simulink model "NavV1_0421_2017a"  (R2017a)
settings: Solver=FixedStepAuto  StartTime=0.0  StopTime=589  FixedStep=dt  RelTol=1e-3
values from neighbouring files (symbols this model uses):
  dt = 0.01    [initNavigation.m]
  g0 = 9.798    [initNavigation.m]
  GPSdt = 0.1    [initNavigation.m]
undefined symbols (not defined in the file or in its folder): DiscIntNeverNeededParam, magnitude, param
libraries: simulink x14, simulink_extras x11, sharedtransform x7, aerolibtransform2 x4, dspstat3 x4, dspsolvers x2, aerolibconvert2 x1
(part 1 of 2)
settings Model: Creator=Ye Xiaoyu  LastModifiedBy=Ye Xiaoyu
settings DataIOCC: ReturnWorkspaceOutputs=on
settings DebuggingCC: SFMachineParentedDataDiag=error
settings SFSimCC: SimUseLocalCustomCode=on
settings RTWCC: RTWUseLocalCustomCode=on

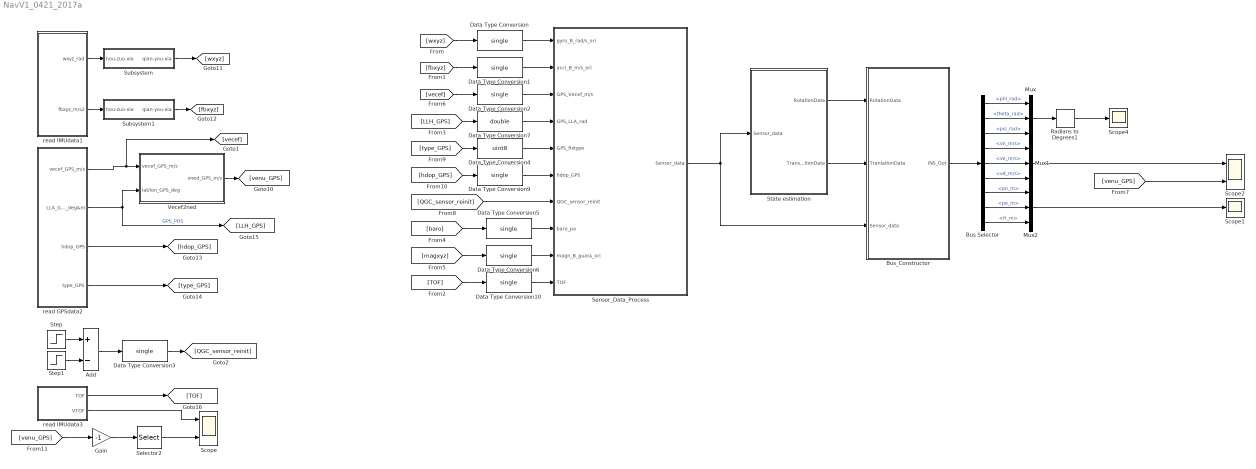
== system NavV1_0421_2017a ==
  Add : Sum  Inputs=+-
  Bus Selector : BusSelector  OutputSignals=phi_rad,theta_rad,psi_rad,vn_m/s,ve_m/s,vd_m/s,pn_m,pe_m,H_m
  Bus_Constructor : Subsystem
  Data Type Conversion{,1..3,5..6,9..10} (8 alike) : DataTypeConversion  OutDataTypeStr=single
  Data Type Conversion4 : DataTypeConversion  OutDataTypeStr=uint8
  Data Type Conversion7 : DataTypeConversion  OutDataTypeStr=double
  Gain : Gain  Gain=-1
  Mux : Mux  Inputs=3
  Mux1 : Mux  Inputs=3
  Mux2 : Mux  Inputs=3
  Radians to Degrees1 : simulink_extras/Transformations/Radians to Degrees
  Scope : Scope  NumInputPorts=2
  Scope1 : Scope
  Scope2 : Scope  NumInputPorts=2
  Scope4 : Scope
  Selector2 : Selector  InputPortWidth=3  IndexOptions=Index vector (dialog)  Indices=[3]  OutputSizes=1
  Sensor_Data_Process : Subsystem
  State estimation : Subsystem
  Step : Step  Time=5  SampleTime=0
  Step1 : Step  Time=5.005  SampleTime=0
  Subsystem : Subsystem
  Subsystem1 : Subsystem
  Vecef2ned : Subsystem
  read GPSdata2 : Subsystem
  read IMUdata1 : Subsystem
  read IMUdata3 : Subsystem
  wires:
  [wxyz] -> Data Type Conversion/1
  [fbxyz] -> Data Type Conversion1/1
  read GPSdata2/1(vecef_GPS_m/s) -> [vecef], Vecef2ned/1(vecef_GPS_m/s)
  [type_GPS] -> Data Type Conversion4/1
  Data Type Conversion/1 -> Sensor_Data_Process/1(gyro_B_rad/s_ori)
  Data Type Conversion1/1 -> Sensor_Data_Process/2(accl_B_m/s_ori)
  Data Type Conversion2/1 -> Sensor_Data_Process/3(GPS_Vecef_m/s)
  [LLH_GPS] -> Data Type Conversion7/1
  Data Type Conversion4/1 -> Sensor_Data_Process/5(GPS_fixtype)
  [QGC_sensor_reinit] -> Sensor_Data_Process/7(QGC_sensor_reinit)
  [baro] -> Data Type Conversion5/1
  [magxyz] -> Data Type Conversion6/1
  Sensor_Data_Process/1(Sensor_data) -> Bus_Constructor/3(Sensor_data), State estimation/1(Sensor_data)
  Data Type Conversion5/1 -> Sensor_Data_Process/8(baro_pa)
  Data Type Conversion6/1 -> Sensor_Data_Process/9(magn_B_guass_ori)
  Data Type Conversion7/1 -> Sensor_Data_Process/4(GPS_LLA_rad)
  Mux1/1 -> Scope2/1
  [venu_GPS] -> Scope2/2
  Mux2/1 -> Scope1/1
  read IMUdata1/2(fbxyz_m/s2) -> Subsystem1/1(hou-zuo-xia)
  read IMUdata1/1(wxyz_rad) -> Subsystem/1(hou-zuo-xia)
  read GPSdata2/2(LLA_GPS_deg&m) -> [LLH_GPS], Vecef2ned/2(lat/lon_GPS_deg)  "GPS_POS"
  Vecef2ned/1(vned_GPS_m/s) -> [venu_GPS]
  read GPSdata2/3(hdop_GPS) -> [hdop_GPS]
  read GPSdata2/4(type_GPS) -> [type_GPS]
  Data Type Conversion9/1 -> Sensor_Data_Process/6(hdop_GPS)
  [hdop_GPS] -> Data Type Conversion9/1
  Subsystem/1(qian-you-xia) -> [wxyz]
  Subsystem1/1(qian-you-xia) -> [fbxyz]
  read IMUdata3/1(TOF) -> [TOF]
  [TOF] -> Data Type Conversion10/1
  Data Type Conversion10/1 -> Sensor_Data_Process/10(TOF)
  read IMUdata3/2(VTOF) -> Scope/1
  [venu_GPS] -> Gain/1
  Selector2/1 -> Scope/2
  Gain/1 -> Selector2/1
  State estimation/1(RotationData) -> Bus_Constructor/1(RotationData)
  State estimation/2(TranslationData) -> Bus_Constructor/2(TranlationData)
  Bus_Constructor/1(INS_Out) -> Bus Selector/1
  Bus Selector/1 -> Mux/1  "<phi_rad>"
  Bus Selector/2 -> Mux/2  "<theta_rad>"
  Bus Selector/3 -> Mux/3  "<psi_rad>"
  Bus Selector/4 -> Mux1/1  "<vn_m/s>"
  Bus Selector/5 -> Mux1/2  "<ve_m/s>"
  Bus Selector/6 -> Mux1/3  "<vd_m/s>"
  Bus Selector/7 -> Mux2/1  "<pn_m>"
  Bus Selector/8 -> Mux2/2  "<pe_m>"
  Bus Selector/9 -> Mux2/3  "<H_m>"
  Mux/1 -> Radians to Degrees1/1
  Radians to Degrees1/1 -> Scope4/1
  [vecef] -> Data Type Conversion2/1
  Step/1 -> Add/1
  Add/1 -> Data Type Conversion3/1
  Step1/1 -> Add/2
  Data Type Conversion3/1 -> [QGC_sensor_reinit]

== system NavV1_0421_2017a/Bus_Constructor ==
  RotationData : Inport
  TranlationData : Inport  Port=2
  Sensor_data : Inport  Port=3
  Bus Creator : BusCreator  Inputs=13
  Bus Selector1 : BusSelector  OutputSignals=vn_m/s,ve_m/s,vd_m/s,pn_m,pe_m,H_m
  Bus Selector2 : BusSelector  OutputSignals=IMU_Data.gyro_B_rad/s_LPF,IMU_Data.accl_B_m/s2_LPF,QGC_sensor_reinit
  Rotation_output : Subsystem
  Signal Copy : SignalConversion  OverrideOpt=off
  Signal Copy2 : SignalConversion  OverrideOpt=off
  INS_Out : Outport
  wires:
  Signal Copy/1 -> Bus Selector2/1
  Sensor_data/1 -> Signal Copy/1
  Bus Selector2/1 -> Bus Creator/1  "<gyro_B_rad/s_LPF>"
  Bus Selector2/2 -> Bus Creator/2  "<accl_B_m/s2_LPF>"
  Bus Selector2/3 -> Bus Creator/3  "<QGC_sensor_reinit>"
  TranlationData/1 -> Signal Copy2/1
  Signal Copy2/1 -> Bus Selector1/1
  Bus Selector1/1 -> Bus Creator/4  "<vn_m/s>"
  Bus Selector1/2 -> Bus Creator/5  "<ve_m/s>"
  Bus Selector1/3 -> Bus Creator/6  "<vd_m/s>"
  Bus Selector1/4 -> Bus Creator/7  "<pn_m>"
  Bus Selector1/5 -> Bus Creator/8  "<pe_m>"
  Bus Selector1/6 -> Bus Creator/9  "<H_m>"
  RotationData/1 -> Rotation_output/1(RotationData)
  Rotation_output/1(<q_update>) -> Bus Creator/10
  Rotation_output/2(phi_rad) -> Bus Creator/11
  Rotation_output/3(theta_rad) -> Bus Creator/12
  Rotation_output/4(psi_rad) -> Bus Creator/13
  Bus Creator/1 -> INS_Out/1

== system NavV1_0421_2017a/Sensor_Data_Process ==
  gyro_B_rad/s_ori : Inport
  accl_B_m/s_ori : Inport  Port=2
  GPS_Vecef_m/s : Inport  Port=3
  GPS_LLA_rad : Inport  Port=4
  GPS_fixtype : Inport  Port=5
  hdop_GPS : Inport  Port=6
  QGC_sensor_reinit : Inport  Port=7
  baro_pa : Inport  Port=8
  magn_B_guass_ori : Inport  Port=9
  TOF : Inport  Port=10
  Bus Creator : BusCreator  Inputs=6
  GPS_Data_Process : Subsystem
  IMU_Data_Process : Subsystem
  Magn_Data_Process : Subsystem
  QGC_sensor_reinit1 : InportShadow  Port=7
  TOF_Data_Process : Subsystem
  baro_Data_Process : Subsystem
  Sensor_data : Outport
  wires:
  QGC_sensor_reinit/1 -> baro_Data_Process/2(QGC_sensor_reinit), GPS_Data_Process/5(QGC_sensor_reinit)  "QGC_sensor_reinit"
  GPS_Data_Process/1(GPS_Data) -> Bus Creator/2  "GPS_Data"
  IMU_Data_Process/1(IMU_Data) -> Bus Creator/1  "IMU_Data"
  baro_Data_Process/1(BARO_Data) -> Bus Creator/3  "BARO_Data"
  gyro_B_rad/s_ori/1 -> IMU_Data_Process/1(gyro_B_rad/s_ori)
  Magn_Data_Process/1(MAGN_Data) -> Bus Creator/4  "MAGN_Data"
  baro_pa/1 -> baro_Data_Process/1(baro)
  accl_B_m/s_ori/1 -> IMU_Data_Process/2(accl_B_m/s_ori)
  magn_B_guass_ori/1 -> Magn_Data_Process/1(magn_B_guass_ori)
  GPS_LLA_rad/1 -> GPS_Data_Process/2(GPS_LLA_rad)
  GPS_Vecef_m/s/1 -> GPS_Data_Process/1(GPS_Vecef_m/s)
  GPS_fixtype/1 -> GPS_Data_Process/3(GPS_fixtype)
  Bus Creator/1 -> Sensor_data/1
  hdop_GPS/1 -> GPS_Data_Process/4(hdop_GPS)
  QGC_sensor_reinit1/1 -> Bus Creator/6  "QGC_sensor_reinit"
  TOF/1 -> TOF_Data_Process/1(TOF_mm_ori)
  TOF_Data_Process/1(TOF_Data) -> Bus Creator/5

== system NavV1_0421_2017a/State estimation ==
  Sensor_data : Inport
  AHRS : Subsystem
  Bus Selector : BusSelector  OutputSignals=QGC_sensor_reinit,IMU_Data.accl_B_m/s2_LPF,MAGN_Data,GPS_Data
  Sensor_data1 : InportShadow
  Sensor_data2 : InportShadow
  Translation_estimate : Subsystem
  RotationData : Outport
  TranslationData : Outport  Port=2
  wires:
  Sensor_data/1 -> Bus Selector/1
  Bus Selector/1 -> AHRS/1(<QGC_sensor_reinit>)  "<QGC_sensor_reinit>"
  Bus Selector/2 -> AHRS/2(<accl_B_m/s2_LPF>)  "<accl_B_m/s2_LPF>"
  Bus Selector/3 -> AHRS/3(<MAGN_Data>)  "<MAGN_Data>"
  Bus Selector/4 -> AHRS/4(<GPS_Data>)  "<GPS_Data>"
  Sensor_data1/1 -> AHRS/5(Sensor_data)
  AHRS/1(RotationData) -> RotationData/1, Translation_estimate/1(RotationData)
  Sensor_data2/1 -> Translation_estimate/2(Sensor_data)
  Translation_estimate/1(TranslationData) -> TranslationData/1

== system NavV1_0421_2017a/Subsystem ==
  hou-zuo-xia : Inport
  Demux : Demux  Outputs=3
  Gain : Gain  Gain=-1
  Gain1 : Gain  Gain=-1
  Mux : Mux  Inputs=3
  qian-you-xia : Outport
  wires:
  Mux/1 -> qian-you-xia/1
  Gain1/1 -> Mux/2
  Demux/3 -> Mux/3
  Gain/1 -> Mux/1
  hou-zuo-xia/1 -> Demux/1
  Demux/1 -> Gain/1
  Demux/2 -> Gain1/1

== system NavV1_0421_2017a/Subsystem1 ==
  hou-zuo-xia : Inport
  Demux : Demux  Outputs=3
  Gain : Gain  Gain=-1
  Gain1 : Gain  Gain=-1
  Mux : Mux  Inputs=3
  qian-you-xia : Outport
  wires:
  Demux/2 -> Gain1/1
  Demux/1 -> Gain/1
  hou-zuo-xia/1 -> Demux/1
  Gain/1 -> Mux/1
  Demux/3 -> Mux/3
  Gain1/1 -> Mux/2
  Mux/1 -> qian-you-xia/1

== system NavV1_0421_2017a/Vecef2ned ==
  vecef_GPS_m/s : Inport
  lat/lon_GPS_deg : Inport  Port=2
  Direction Cosine Matrix ECEF to NED : aerolibtransform2/Direction Cosine Matrix ECEF to NED
      settings: SourceProductBaseCode=AE
  Product : Product  Multiplication=Matrix(*)
  Radians to Degrees : simulink_extras/Transformations/Radians to Degrees
  Selector2 : Selector  InputPortWidth=3  IndexOptions=Index vector (dialog)  Indices=[1 2]  OutputSizes=1
  vned_GPS_m/s : Outport
  wires:
  Direction Cosine Matrix ECEF to NED/1 -> Product/1
  vecef_GPS_m/s/1 -> Product/2
  lat/lon_GPS_deg/1 -> Selector2/1
  Product/1 -> vned_GPS_m/s/1
  Selector2/1 -> Radians to Degrees/1
  Radians to Degrees/1 -> Direction Cosine Matrix ECEF to NED/1

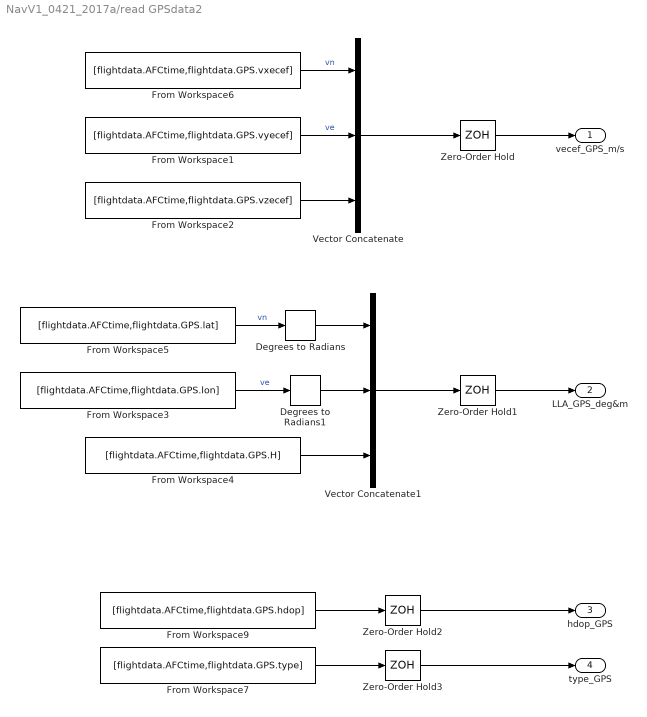
== system NavV1_0421_2017a/read GPSdata2 ==
  Degrees to Radians : simulink_extras/Transformations/Degrees to Radians
  Degrees to Radians1 : simulink_extras/Transformations/Degrees to Radians
  From Workspace1 : FromWorkspace  VariableName=[flightdata.AFCtime,flightdata.GPS.vyecef]
  From Workspace2 : FromWorkspace  VariableName=[flightdata.AFCtime,flightdata.GPS.vzecef]
  From Workspace3 : FromWorkspace  VariableName=[flightdata.AFCtime,flightdata.GPS.lon]
  From Workspace4 : FromWorkspace  VariableName=[flightdata.AFCtime,flightdata.GPS.H]
  From Workspace5 : FromWorkspace  VariableName=[flightdata.AFCtime,flightdata.GPS.lat]
  From Workspace6 : FromWorkspace  VariableName=[flightdata.AFCtime,flightdata.GPS.vxecef]
  From Workspace7 : FromWorkspace  VariableName=[flightdata.AFCtime,flightdata.GPS.type]
  From Workspace9 : FromWorkspace  VariableName=[flightdata.AFCtime,flightdata.GPS.hdop]
  Vector Concatenate : Concatenate  NumInputs=3
  Vector Concatenate1 : Concatenate  NumInputs=3
  Zero-Order Hold{,1..3} (4 alike) : ZeroOrderHold  SampleTime=GPSdt
  vecef_GPS_m/s : Outport
  LLA_GPS_deg&m : Outport  Port=2
  hdop_GPS : Outport  Port=3
  type_GPS : Outport  Port=4
  wires:
  Zero-Order Hold/1 -> vecef_GPS_m/s/1
  Zero-Order Hold1/1 -> LLA_GPS_deg&m/1
  From Workspace6/1 -> Vector Concatenate/1  "vn"
  From Workspace1/1 -> Vector Concatenate/2  "ve"
  From Workspace2/1 -> Vector Concatenate/3
  From Workspace5/1 -> Degrees to Radians/1  "vn"
  From Workspace3/1 -> Degrees to Radians1/1  "ve"
  From Workspace4/1 -> Vector Concatenate1/3
  Vector Concatenate/1 -> Zero-Order Hold/1
  Vector Concatenate1/1 -> Zero-Order Hold1/1
  From Workspace7/1 -> Zero-Order Hold3/1
  Zero-Order Hold2/1 -> hdop_GPS/1
  From Workspace9/1 -> Zero-Order Hold2/1
  Zero-Order Hold3/1 -> type_GPS/1
  Degrees to Radians/1 -> Vector Concatenate1/1
  Degrees to Radians1/1 -> Vector Concatenate1/2

== system NavV1_0421_2017a/read IMUdata1 ==
  note: 后-左-下
  Degrees to Radians1 : simulink_extras/Transformations/Degrees to Radians
  From Workspace1 : FromWorkspace  VariableName=[flightdata.AFCtime,flightdata.IMUADIS16507.wx]
  From Workspace10 : FromWorkspace  VariableName=[flightdata.AFCtime,flightdata.IMUADIS16507.wy]
  From Workspace2 : FromWorkspace  VariableName=[flightdata.AFCtime,flightdata.IMUADIS16507.wz]
  From Workspace3 : FromWorkspace  VariableName=[flightdata.AFCtime,flightdata.IMUADIS16507.fbx]
  From Workspace4 : FromWorkspace  VariableName=[flightdata.AFCtime,flightdata.IMUADIS16507.fby]
  From Workspace5 : FromWorkspace  VariableName=[flightdata.AFCtime,flightdata.IMUADIS16507.fbz]
  Scope : Scope
  Vector Concatenate : Concatenate  NumInputs=3
  Vector Concatenate1 : Concatenate  NumInputs=3
  Zero-Order Hold : ZeroOrderHold  SampleTime=dt
  Zero-Order Hold1 : ZeroOrderHold  SampleTime=dt
  wxyz_rad : Outport
  fbxyz_m/s2 : Outport  Port=2
  wires:
  Degrees to Radians1/1 -> Zero-Order Hold/1
  Zero-Order Hold1/1 -> fbxyz_m/s2/1
  Zero-Order Hold/1 -> wxyz_rad/1
  From Workspace1/1 -> Vector Concatenate/1
  From Workspace10/1 -> Vector Concatenate/2
  From Workspace2/1 -> Vector Concatenate/3
  Vector Concatenate/1 -> Scope/1, Degrees to Radians1/1
  From Workspace3/1 -> Vector Concatenate1/1
  From Workspace4/1 -> Vector Concatenate1/2
  From Workspace5/1 -> Vector Concatenate1/3
  Vector Concatenate1/1 -> Zero-Order Hold1/1

== system NavV1_0421_2017a/read IMUdata3 ==
  note: 后-左-下
  Data Type Conversion : DataTypeConversion  OutDataTypeStr=single
  From Workspace1 : FromWorkspace  VariableName=[flightdata.AFCtime,flightdata.TOF.dist]
  From Workspace10 : FromWorkspace  VariableName=[flightdata.AFCtime,flightdata.TOF.Inten]
  From Workspace2 : FromWorkspace  VariableName=[flightdata.AFCtime,flightdata.TOF.sts]
  Gain : Gain  Gain=0.01
  Scope : Scope
  Scope1 : Scope  NumInputPorts=3
  TD_baro : Subsystem
  Vector Concatenate : Concatenate  NumInputs=3
  Zero-Order Hold : ZeroOrderHold  SampleTime=dt
  TOF : Outport
  VTOF : Outport  Port=2
  wires:
  Vector Concatenate/1 -> Zero-Order Hold/1, Scope/1
  From Workspace2/1 -> Vector Concatenate/3
  From Workspace10/1 -> Vector Concatenate/2
  From Workspace1/1 -> Scope1/1, Data Type Conversion/1, Vector Concatenate/1
  Zero-Order Hold/1 -> TOF/1
  TD_baro/1(vH_baro_TD) -> VTOF/1, Scope1/2  "vH_baro_m/s_TD"
  TD_baro/2(H_baro_TD) -> Scope1/3  "H_baro_TD"
  Data Type Conversion/1 -> Gain/1
  Gain/1 -> TD_baro/1(H_baro)

== system NavV1_0421_2017a/Bus_Constructor/Rotation_output ==
  RotationData : Inport
  Bus Selector3 : BusSelector  OutputSignals=q_update
  Data Type Conversion11 : DataTypeConversion  OutDataTypeStr=single
  Data Type Conversion12 : DataTypeConversion  OutDataTypeStr=double
  Demux : Demux  Outputs=3
  Quaternions to Rotation Angles1 : sharedtransform/Quaternions to Rotation Angles  rotationOrder=ZYX
      settings: SourceProductBaseCode=AE,PW,DR,MT,UV,VE
  Signal Copy1 : SignalConversion  OverrideOpt=off
  <q_update> : Outport
  phi_rad : Outport  Port=2
  theta_rad : Outport  Port=3
  psi_rad : Outport  Port=4
  wires:
  Quaternions to Rotation Angles1/1 -> Data Type Conversion11/1
  Bus Selector3/1 -> <q_update>/1, Data Type Conversion12/1  "<q_update>"
  Signal Copy1/1 -> Bus Selector3/1
  RotationData/1 -> Signal Copy1/1
  Data Type Conversion12/1 -> Quaternions to Rotation Angles1/1
  Demux/1 -> psi_rad/1  "psi_rad"
  Data Type Conversion11/1 -> Demux/1
  Demux/2 -> theta_rad/1  "theta_rad"
  Demux/3 -> phi_rad/1  "phi_rad"

== system NavV1_0421_2017a/Sensor_Data_Process/GPS_Data_Process ==
  note: GPS_fixtype:
      | 0: 定位不可用或无效
      | 1:单点定位
      | 2:伪距差分
      | 4:RTK固定解
  GPS_Vecef_m/s : Inport
  GPS_LLA_rad : Inport  Port=2
  GPS_fixtype : Inport  Port=3
  hdop_GPS : Inport  Port=4
  QGC_sensor_reinit : Inport  Port=5
  Bus Creator : BusCreator  Inputs=13
  Demux : Demux  Outputs=3
  Demux1 : Demux  Outputs=3
  Demux3 : Demux  Outputs=3
  LLA2NED : Subsystem
  Subsystem : Subsystem
  GPS_Data : Outport
  wires:
  Bus Creator/1 -> GPS_Data/1
  Demux3/3 -> Bus Creator/3  "H_gps"
  Demux/3 -> Bus Creator/9  "vd_gps"
  Demux/1 -> Bus Creator/7  "vn_gps"
  GPS_LLA_rad/1 -> Demux3/1, LLA2NED/1(gps_LLA_rad)
  Demux/2 -> Bus Creator/8  "ve_gps"
  Demux3/2 -> Bus Creator/2  "lon_gps"
  Demux3/1 -> Bus Creator/1  "lat_gps"
  GPS_fixtype/1 -> Bus Creator/12  "fixtype_gps"
  QGC_sensor_reinit/1 -> LLA2NED/3(QGC_sensor_reinit)  "QGC_sensor_reinit"
  LLA2NED/1("gpsposNEDout ") -> Demux1/1
  Demux1/1 -> Bus Creator/4  "pos_N_gps"
  Demux1/2 -> Bus Creator/5  "pos_E_gps"
  Demux1/3 -> Bus Creator/6  "pos_D_gps"
  GPS_Vecef_m/s/1 -> LLA2NED/2(GPS_Vecef_m/s)
  LLA2NED/2(gpsvNEDout) -> Subsystem/1(Vned), Demux/1
  Subsystem/1(heading_GPS_rad) -> Bus Creator/10  "heading_GPS_rad"
  Subsystem/2(heading_GPS_valid) -> Bus Creator/11  "heading_GPS_valid"
  hdop_GPS/1 -> Bus Creator/13  "hdop_GPS"

== system NavV1_0421_2017a/Sensor_Data_Process/IMU_Data_Process ==
  gyro_B_rad/s_ori : Inport
  accl_B_m/s_ori : Inport  Port=2
  Bus Creator : BusCreator  Inputs=2
  accl_preprocessing : Subsystem
  gyro_preprocessing : Subsystem
  IMU_Data : Outport  PortDimensions=6
  wires:
  Bus Creator/1 -> IMU_Data/1
  gyro_preprocessing/1(gyro_B_rad/s_LPF) -> Bus Creator/1  "gyro_B_rad/s_LPF"
  accl_B_m/s_ori/1 -> accl_preprocessing/1(accl_B_m/s_ori)
  accl_preprocessing/1(accl_B_m/s2_LPF) -> Bus Creator/2  "accl_B_m/s2_LPF"
  gyro_B_rad/s_ori/1 -> gyro_preprocessing/1(gyro_B_rad/s_ori)

== system NavV1_0421_2017a/Sensor_Data_Process/Magn_Data_Process ==
  magn_B_guass_ori : Inport
  gyro_preprocessing : Subsystem
  MAGN_Data : Outport
  wires:
  magn_B_guass_ori/1 -> gyro_preprocessing/1(gyro_B_rad/s_ori)
  gyro_preprocessing/1(gyro_B_rad/s_LPF) -> MAGN_Data/1  "gyro_B_rad/s_LPF"

== system NavV1_0421_2017a/Sensor_Data_Process/TOF_Data_Process ==
  TOF_mm_ori : Inport
  Bus Creator1 : BusCreator  Inputs=4
  Data Type Conversion : DataTypeConversion  OutDataTypeStr=uint8
  Demux : Demux  Outputs=3
  Gain : Gain  Gain=0.01
  TD_baro : Subsystem
  TOF_Data : Outport
  wires:
  TD_baro/2(H_TOF_TD) -> Bus Creator1/2  "H_TOF_TD"
  Demux/3 -> Data Type Conversion/1  "TOF_sts"
  Demux/1 -> Gain/1
  TOF_mm_ori/1 -> Demux/1
  Demux/2 -> Bus Creator1/3  "TOF_Inten"
  Bus Creator1/1 -> TOF_Data/1  "TOF_Data"
  TD_baro/1(vH_TOF_TD) -> Bus Creator1/1  "vH_TOF_m/s_TD"
  Gain/1 -> TD_baro/1(H_TOF)  "TOF_Dist_m"
  Data Type Conversion/1 -> Bus Creator1/4  "TOF_sts"

== system NavV1_0421_2017a/Sensor_Data_Process/baro_Data_Process ==
  baro : Inport
  QGC_sensor_reinit : Inport  Port=2
  Bus Creator : BusCreator  Inputs=2
  Pressure2Height : Subsystem
  Scope : Scope  NumInputPorts=2
  Sum : Sum  Inputs=|+-
  TD_baro : Subsystem
  reinit_baro0 : Subsystem
  BARO_Data : Outport  PortDimensions=2
  wires:
  Sum/1 -> Bus Creator/2  "H_baro_m_TD"
  TD_baro/1(vH_baro_TD) -> Scope/1, Bus Creator/1  "vH_baro_m/s_TD"
  baro/1 -> Pressure2Height/1(baro)
  Bus Creator/1 -> BARO_Data/1
  Pressure2Height/1(H_baro) -> TD_baro/1(H_baro)
  QGC_sensor_reinit/1 -> reinit_baro0/1(QGC_sensor_reinit)
  TD_baro/2(H_baro_TD) -> Scope/2, Sum/1, reinit_baro0/2(Data)  "H_baro_TD"
  reinit_baro0/1(dataout) -> Sum/2

== system NavV1_0421_2017a/State estimation/AHRS ==
  <QGC_sensor_reinit> : Inport  PortDimensions=1
  <accl_B_m/s2_LPF> : Inport  Port=2  PortDimensions=3
  <MAGN_Data> : Inport  Port=3  PortDimensions=3
  <GPS_Data> : Inport  Port=4
  Sensor_data : Inport  Port=5
  <QGC_sensor_reinit>1 : InportShadow  PortDimensions=1
  AHRS Complementary filter : Subsystem  mask{GPS_accel_kp=0.2, GPS_accel_ki=0, noGPS_accel_kp=0.3, noGPS_accel_ki=0}
      mask prompts: GPS_accel_kp "GPS修正下互补滤波增益kp"; GPS_accel_ki "GPS修正下互补滤波增益Ki"; noGPS_accel_kp "无GPS修正下互补滤波增益kp"; noGPS_accel_ki "无GPS修正下互补滤波增益Ki"
      mask DialogControl DescTextVar Prompt: AHRS Complementary filter
  Bus Selector1 : BusSelector  OutputSignals=IMU_Data.accl_B_m/s2_LPF
  Bus Selector2 : BusSelector  OutputSignals=MAGN_Data
  Init_Q0 : Subsystem
  Scope : Scope
  Sensor_data_1 : InportShadow  Port=5
  att_update : Subsystem
  RotationData : Outport
  wires:
  Sensor_data/1 -> att_update/1(Sensor_data)
  Sensor_data_1/1 -> Bus Selector2/1, Bus Selector1/1
  Bus Selector1/1 -> AHRS Complementary filter/1(fbxyz)  "<accl_B_m/s2_LPF>"
  Bus Selector2/1 -> AHRS Complementary filter/4(magxyz)  "<MAGN_Data>"
  <GPS_Data>/1 -> AHRS Complementary filter/3(GPS_Data)
  <QGC_sensor_reinit>1/1 -> att_update/3(init_flag)
  att_update/1(att_update) -> RotationData/1, AHRS Complementary filter/2(Q_update)
  AHRS Complementary filter/1(w_bias) -> att_update/4(wbias), Scope/1
  <QGC_sensor_reinit>/1 -> Init_Q0/1(U)
  <accl_B_m/s2_LPF>/1 -> Init_Q0/2(accl_B_m/s_LPF)
  <MAGN_Data>/1 -> Init_Q0/3(Magn_B_guess_LPF)
  Init_Q0/1(quat_0) -> att_update/2(quat_0)

== system NavV1_0421_2017a/State estimation/Translation_estimate ==
  RotationData : Inport
  Sensor_data : Inport  Port=2
  Bus Creator : BusCreator  Inputs=2
  Bus Creator2 : BusCreator  Inputs=6
  Demux : Demux  Outputs=2
  Demux1 : Demux  Outputs=2
  Gain : Gain  Gain=-1
  High data source selection : Subsystem
  Rxy_Horizontal_estimation : Subsystem
  Subsystem : Subsystem
  V_Horizontal_estimation : Subsystem
  V_Vertical_estimation : Subsystem
  translate to N : Subsystem
  TranslationData : Outport
  wires:
  Sensor_data/1 -> High data source selection/1(Sensor_data), Subsystem/2(sensor_data), V_Vertical_estimation/2(Sensor_data), Rxy_Horizontal_estimation/3(Sensor_data2), V_Horizontal_estimation/2(Sensor_data2), translate to N/2(Sensor_data)
  RotationData/1 -> translate to N/1(RotationData)
  Rxy_Horizontal_estimation/1(R_n&e) -> Demux1/1
  translate to N/1(accel_Horizontal_predict) -> V_Horizontal_estimation/1(An)
  V_Horizontal_estimation/1(vxy_estimout) -> Demux/1  "v_ne_"
  V_Horizontal_estimation/2(V_n&e) -> Rxy_Horizontal_estimation/1(Vn)
  V_Horizontal_estimation/3(GPS_v_enable) -> Rxy_Horizontal_estimation/2(Enable)
  translate to N/2(accel_Vertical_predict) -> V_Vertical_estimation/1(accel_Vertical_predict)
  V_Vertical_estimation/1(Vh_vertical_eastimate) -> Subsystem/1(Vh_vertical_eastimate), Gain/1  "vh_m/s"
  High data source selection/1(HTOF_vaild_flag) -> Bus Creator/1  "HTOF_vaild"
  High data source selection/2(HGPS_vaild_flag) -> Bus Creator/2  "HGPS_vaild"
  Bus Creator/1 -> Subsystem/3(Vertical_vaild_flag), V_Vertical_estimation/3(Vertical_vaild_flag)
  Subsystem/1(H_estimation) -> Bus Creator2/6  "H_m"
  Demux/1 -> Bus Creator2/1  "vn_m/s"
  Demux/2 -> Bus Creator2/2  "ve_m/s"
  Demux1/1 -> Bus Creator2/4  "pn_m"
  Demux1/2 -> Bus Creator2/5  "pe_m"
  Gain/1 -> Bus Creator2/3  "vd_m/s"
  Bus Creator2/1 -> TranslationData/1

== system NavV1_0421_2017a/read IMUdata3/TD_baro ==
  H_baro : Inport
  Constant1 : Constant  Value=dt  OutDataTypeStr=single
  Constant3 : Constant  Value=0.23  OutDataTypeStr=single
  Constant4 : Constant  Value=1000  OutDataTypeStr=single
  Delay1 : Delay  DelayLength=1  InitialConditionSource=Input port
      settings: InputPortMap=u0,p4
  MATLAB Function2 : MATLAB Function  TreatAsAtomicUnit=on
  Memory : Memory  InheritSampleTime=on
  Scope : Scope  NumInputPorts=3
  vH_baro_TD : Outport
  H_baro_TD : Outport  Port=2
  wires:
  Delay1/1 -> H_baro_TD/1, Scope/3, MATLAB Function2/3("u1 ")
  H_baro/1 -> Delay1/2, MATLAB Function2/2(u0), Scope/1
  Memory/1 -> MATLAB Function2/4("u2 "), vH_baro_TD/1, Scope/2
  Constant3/1 -> MATLAB Function2/5(h)
  Constant1/1 -> MATLAB Function2/1(T)
  Constant4/1 -> MATLAB Function2/6(r)
  MATLAB Function2/1(u1) -> Delay1/1
  MATLAB Function2/2(u2) -> Memory/1

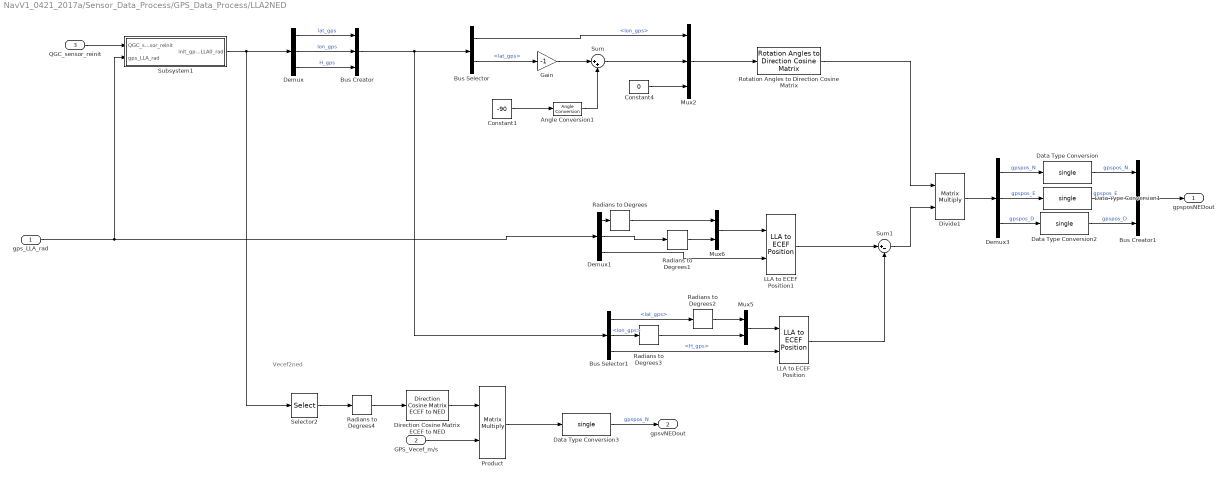
== system NavV1_0421_2017a/Sensor_Data_Process/GPS_Data_Process/LLA2NED ==
  note: Vecef2ned
  gps_LLA_rad : Inport
  GPS_Vecef_m/s : Inport  Port=2
  QGC_sensor_reinit : Inport  Port=3
  Angle Conversion1 : aerolibconvert2/Angle Conversion  IU=deg  OU=rad
  Bus Creator : BusCreator  Inputs=3
  Bus Creator1 : BusCreator  Inputs=3
  Bus Selector : BusSelector  OutputSignals=lon_gps,lat_gps
  Bus Selector1 : BusSelector  OutputSignals=lat_gps,lon_gps,H_gps
  Constant1 : Constant  Value=-90
  Constant4 : Constant  Value=0
  Data Type Conversion{,1..3} (4 alike) : DataTypeConversion  OutDataTypeStr=single
  Demux : Demux  Outputs=3
  Demux1 : Demux  Outputs=3
  Demux3 : Demux  Outputs=3
  Direction Cosine Matrix ECEF to NED : aerolibtransform2/Direction Cosine Matrix ECEF to NED
      settings: SourceProductBaseCode=AE
  Divide1 : Product  Inputs=**  Multiplication=Matrix(*)
  Gain : Gain  Gain=-1
  LLA to ECEF Position : aerolibtransform2/LLA to ECEF Position  R=6378137
  LLA to ECEF Position1 : aerolibtransform2/LLA to ECEF Position  R=6378137
  Mux2 : Mux  Inputs=3
  Mux5 : Mux  Inputs=2
  Mux6 : Mux  Inputs=2
  Product : Product  Multiplication=Matrix(*)
  Radians to Degrees{,1..4} (5 alike) : simulink_extras/Transformations/Radians to Degrees
  Rotation Angles to Direction Cosine Matrix : sharedtransform/Rotation Angles to Direction Cosine Matrix  rotationOrder=ZYX
      settings: SourceProductBaseCode=AE
  Selector2 : Selector  InputPortWidth=3  IndexOptions=Index vector (dialog)  Indices=[1 2]  OutputSizes=1
  Subsystem1 : Subsystem
  Sum : Sum  Inputs=|++
  Sum1 : Sum  Inputs=|+-
  "gpsposNEDout " : Outport
  gpsvNEDout : Outport  Port=2
  wires:
  Bus Creator1/1 -> "gpsposNEDout "/1
  Demux3/3 -> Data Type Conversion2/1  "gpspos_D"
  Demux3/2 -> Data Type Conversion1/1  "gpspos_E"
  Demux3/1 -> Data Type Conversion/1  "gpspos_N"
  Bus Creator/1 -> Bus Selector/1, Bus Selector1/1
  Demux/3 -> Bus Creator/3  "H_gps"
  Demux/2 -> Bus Creator/2  "lon_gps"
  Demux/1 -> Bus Creator/1  "lat_gps"
  Demux1/3 -> LLA to ECEF Position1/2
  Mux6/1 -> LLA to ECEF Position1/1
  Mux5/1 -> LLA to ECEF Position/1
  Gain/1 -> Sum/1
  LLA to ECEF Position1/1 -> Sum1/1
  Constant4/1 -> Mux2/3
  Sum1/1 -> Divide1/2
  Divide1/1 -> Demux3/1
  Demux1/1 -> Radians to Degrees/1
  Mux2/1 -> Rotation Angles to Direction Cosine Matrix/1
  Rotation Angles to Direction Cosine Matrix/1 -> Divide1/1
  Constant1/1 -> Angle Conversion1/1
  LLA to ECEF Position/1 -> Sum1/2
  Demux1/2 -> Radians to Degrees1/1
  Sum/1 -> Mux2/2
  Bus Selector/2 -> Gain/1  "<lat_gps>"
  Bus Selector/1 -> Mux2/1  "<lon_gps>"
  Bus Selector1/1 -> Radians to Degrees2/1  "<lat_gps>"
  Bus Selector1/2 -> Radians to Degrees3/1  "<lon_gps>"
  Bus Selector1/3 -> LLA to ECEF Position/2  "<H_gps>"
  gps_LLA_rad/1 -> Subsystem1/2(gps_LLA_rad), Demux1/1
  Radians to Degrees/1 -> Mux6/1
  Radians to Degrees1/1 -> Mux6/2
  QGC_sensor_reinit/1 -> Subsystem1/1(QGC_sensor_reinit)
  Data Type Conversion/1 -> Bus Creator1/1  "gpspos_N"
  Data Type Conversion1/1 -> Bus Creator1/2  "gpspos_E"
  Data Type Conversion2/1 -> Bus Creator1/3  "gpspos_D"
  Angle Conversion1/1 -> Sum/2
  Radians to Degrees2/1 -> Mux5/1
  Radians to Degrees3/1 -> Mux5/2
  Product/1 -> Data Type Conversion3/1
  Subsystem1/1(init_gps_LLA0_rad) -> Selector2/1, Demux/1
  GPS_Vecef_m/s/1 -> Product/2
  Direction Cosine Matrix ECEF to NED/1 -> Product/1
  Selector2/1 -> Radians to Degrees4/1
  Radians to Degrees4/1 -> Direction Cosine Matrix ECEF to NED/1
  Data Type Conversion3/1 -> gpsvNEDout/1  "gpspos_N"

== system NavV1_0421_2017a/Sensor_Data_Process/GPS_Data_Process/Subsystem ==
  Vned : Inport
  Atan2 : Trigonometry  Operator=atan2
  Compare To Constant : simulink/Logic and Bit Operations/Compare To Constant  relop=>=  const=0.8  OutDataTypeStr=boolean
  Math Function : Math  Operator=magnitude^2  SaturateOnIntegerOverflow=on
  Moving Average : dspstat3/Moving Average  Method=Sliding window  SpecifyWindowLength=on  WindowLength=10  ForgettingFactor=0.9  SimulateUsing=Code generation
  Rate Transition : RateTransition  OutPortSampleTime=GPSdt
  Scope : Scope  NumInputPorts=2
  Scope1 : Scope
  Selector2 : Selector  InputPortWidth=3  IndexOptions=Index vector (dialog)  Indices=[2]  OutputSizes=1
  Selector3 : Selector  InputPortWidth=3  IndexOptions=Index vector (dialog)  Indices=[1]  OutputSizes=1
  Selector4 : Selector  InputPortWidth=3  IndexOptions=Index vector (dialog)  Indices=[1 2]  OutputSizes=1
  Sqrt : Sqrt  SaturateOnIntegerOverflow=on
  Sum of Elements : Sum  Inputs=+
  heading_GPS_rad : Outport
  heading_GPS_valid : Outport  Port=2
  wires:
  Selector2/1 -> Atan2/1
  Math Function/1 -> Sum of Elements/1
  Vned/1 -> Selector2/1, Selector4/1, Selector3/1
  Selector3/1 -> Atan2/2
  Sum of Elements/1 -> Sqrt/1
  Selector4/1 -> Math Function/1
  Sqrt/1 -> Compare To Constant/1
  Compare To Constant/1 -> Scope1/1, heading_GPS_valid/1
  Moving Average/1 -> Scope/2, heading_GPS_rad/1
  Atan2/1 -> Rate Transition/1
  Rate Transition/1 -> Moving Average/1, Scope/1

== system NavV1_0421_2017a/Sensor_Data_Process/IMU_Data_Process/accl_preprocessing ==
  note: front-right-dowm
  accl_B_m/s_ori : Inport
  Constant2 : Constant  Value=1/dt  OutDataTypeStr=single
  Constant4 : Constant  Value=1/dt  OutDataTypeStr=single
  Constant6 : Constant  Value=1/dt  OutDataTypeStr=single
  Constant7 : Constant  Value=param.proces.imu_gyro_cutoff_freq  OutDataTypeStr=single
  Demux : Demux  Outputs=3
  MATLAB Function1 : MATLAB Function  TreatAsAtomicUnit=on
  MATLAB Function2 : MATLAB Function  TreatAsAtomicUnit=on
  MATLAB Function3 : MATLAB Function  TreatAsAtomicUnit=on
  Vector Concatenate : Concatenate  NumInputs=3
  accl_B_m/s2_LPF : Outport
  wires:
  Vector Concatenate/1 -> accl_B_m/s2_LPF/1
  Constant4/1 -> MATLAB Function2/2(sample_freq)
  Constant2/1 -> MATLAB Function1/2(sample_freq)
  accl_B_m/s_ori/1 -> Demux/1
  Demux/1 -> MATLAB Function2/1(curr_input)
  Demux/2 -> MATLAB Function1/1(curr_input)
  Constant6/1 -> MATLAB Function3/2(sample_freq)
  Demux/3 -> MATLAB Function3/1(curr_input)
  Constant7/1 -> MATLAB Function2/3(cutoff_freq), MATLAB Function3/3(cutoff_freq), MATLAB Function1/3(cutoff_freq)
  MATLAB Function3/1(curr_output) -> Vector Concatenate/3  "wz"
  MATLAB Function1/1(curr_output) -> Vector Concatenate/2  "wy"
  MATLAB Function2/1(curr_output) -> Vector Concatenate/1  "wx"

== system NavV1_0421_2017a/Sensor_Data_Process/IMU_Data_Process/gyro_preprocessing ==
  note: front-right-dowm
  note: rad/s
  gyro_B_rad/s_ori : Inport
  Constant2 : Constant  Value=1/dt  OutDataTypeStr=single
  Constant4 : Constant  Value=1/dt  OutDataTypeStr=single
  Constant6 : Constant  Value=1/dt  OutDataTypeStr=single
  Constant7 : Constant  Value=param.proces.imu_gyro_cutoff_freq  OutDataTypeStr=single
  Demux : Demux  Outputs=3
  MATLAB Function1 : MATLAB Function  TreatAsAtomicUnit=on
  MATLAB Function2 : MATLAB Function  TreatAsAtomicUnit=on
  MATLAB Function3 : MATLAB Function  TreatAsAtomicUnit=on
  Scope : Scope  NumInputPorts=2
  Vector Concatenate : Concatenate  NumInputs=3
  gyro_B_rad/s_LPF : Outport
  wires:
  MATLAB Function2/1(curr_output) -> Vector Concatenate/1  "wx"
  MATLAB Function1/1(curr_output) -> Vector Concatenate/2  "wy"
  MATLAB Function3/1(curr_output) -> Vector Concatenate/3  "wz"
  Constant7/1 -> MATLAB Function3/3(cutoff_freq), MATLAB Function1/3(cutoff_freq), MATLAB Function2/3(cutoff_freq)
  Demux/3 -> MATLAB Function3/1(curr_input)
  Constant6/1 -> MATLAB Function3/2(sample_freq)
  Demux/2 -> MATLAB Function1/1(curr_input)
  Demux/1 -> MATLAB Function2/1(curr_input), Scope/2
  gyro_B_rad/s_ori/1 -> Demux/1
  Constant2/1 -> MATLAB Function1/2(sample_freq)
  Constant4/1 -> MATLAB Function2/2(sample_freq)
  Vector Concatenate/1 -> gyro_B_rad/s_LPF/1

== system NavV1_0421_2017a/Sensor_Data_Process/Magn_Data_Process/gyro_preprocessing ==
  note: rad/s
  note: front-right-dowm
  gyro_B_rad/s_ori : Inport
  Constant2 : Constant  Value=1/dt  OutDataTypeStr=single
  Constant4 : Constant  Value=1/dt  OutDataTypeStr=single
  Constant6 : Constant  Value=1/dt  OutDataTypeStr=single
  Constant7 : Constant  Value=param.proces.imu_gyro_cutoff_freq  OutDataTypeStr=single
  Demux : Demux  Outputs=3
  MATLAB Function1 : MATLAB Function  TreatAsAtomicUnit=on
  MATLAB Function2 : MATLAB Function  TreatAsAtomicUnit=on
  MATLAB Function3 : MATLAB Function  TreatAsAtomicUnit=on
  Scope : Scope  NumInputPorts=2
  Vector Concatenate : Concatenate  NumInputs=3
  gyro_B_rad/s_LPF : Outport
  wires:
  Vector Concatenate/1 -> gyro_B_rad/s_LPF/1
  Constant4/1 -> MATLAB Function2/2(sample_freq)
  Constant2/1 -> MATLAB Function1/2(sample_freq)
  gyro_B_rad/s_ori/1 -> Demux/1
  Demux/1 -> Scope/2, MATLAB Function2/1(curr_input)
  Demux/2 -> MATLAB Function1/1(curr_input)
  Constant6/1 -> MATLAB Function3/2(sample_freq)
  Demux/3 -> MATLAB Function3/1(curr_input)
  Constant7/1 -> MATLAB Function2/3(cutoff_freq), MATLAB Function1/3(cutoff_freq), MATLAB Function3/3(cutoff_freq)
  MATLAB Function3/1(curr_output) -> Vector Concatenate/3  "wz"
  MATLAB Function1/1(curr_output) -> Vector Concatenate/2  "wy"
  MATLAB Function2/1(curr_output) -> Vector Concatenate/1  "wx"

== system NavV1_0421_2017a/Sensor_Data_Process/TOF_Data_Process/TD_baro ==
  H_TOF : Inport
  Constant1 : Constant  Value=dt  OutDataTypeStr=single
  Constant3 : Constant  Value=0.23  OutDataTypeStr=single
  Constant4 : Constant  Value=1000  OutDataTypeStr=single
  Delay1 : Delay  DelayLength=1  InitialConditionSource=Input port
      settings: InputPortMap=u0,p4
  MATLAB Function2 : MATLAB Function  TreatAsAtomicUnit=on
  Memory : Memory  InheritSampleTime=on
  Scope : Scope  NumInputPorts=3
  vH_TOF_TD : Outport
  H_TOF_TD : Outport  Port=2
  wires:
  Delay1/1 -> H_TOF_TD/1, Scope/3, MATLAB Function2/3("u1 ")
  H_TOF/1 -> Delay1/2, MATLAB Function2/2(u0), Scope/1
  Memory/1 -> MATLAB Function2/4("u2 "), vH_TOF_TD/1, Scope/2
  Constant3/1 -> MATLAB Function2/5(h)
  Constant1/1 -> MATLAB Function2/1(T)
  Constant4/1 -> MATLAB Function2/6(r)
  MATLAB Function2/1(u1) -> Delay1/1
  MATLAB Function2/2(u2) -> Memory/1

== system NavV1_0421_2017a/Sensor_Data_Process/baro_Data_Process/Pressure2Height ==
  baro : Inport
  Add : Sum  Inputs=+-
  Constant : Constant  OutDataTypeStr=single
  Constant1 : Constant  Value=1/5.255  OutDataTypeStr=single
  Gain : Gain  Gain=1/1.01325
  Gain1 : Gain  Gain=44330
  Math Function : Math  Operator=pow  SaturateOnIntegerOverflow=on
  H_baro : Outport
  wires:
  Gain/1 -> Math Function/1
  Constant1/1 -> Math Function/2
  Math Function/1 -> Add/2
  Constant/1 -> Add/1
  Add/1 -> Gain1/1
  Gain1/1 -> H_baro/1
  baro/1 -> Gain/1

== system NavV1_0421_2017a/Sensor_Data_Process/baro_Data_Process/TD_baro ==
  H_baro : Inport
  Constant1 : Constant  Value=dt  OutDataTypeStr=single
  Constant3 : Constant  Value=0.23  OutDataTypeStr=single
  Constant4 : Constant  Value=1000  OutDataTypeStr=single
  Delay1 : Delay  DelayLength=1  InitialConditionSource=Input port
      settings: InputPortMap=u0,p4
  MATLAB Function2 : MATLAB Function  TreatAsAtomicUnit=on
  Memory : Memory  InheritSampleTime=on
  Scope : Scope  NumInputPorts=3
  vH_baro_TD : Outport
  H_baro_TD : Outport  Port=2
  wires:
  Delay1/1 -> H_baro_TD/1, Scope/3, MATLAB Function2/3("u1 ")
  H_baro/1 -> Delay1/2, MATLAB Function2/2(u0), Scope/1
  Memory/1 -> MATLAB Function2/4("u2 "), vH_baro_TD/1, Scope/2
  Constant3/1 -> MATLAB Function2/5(h)
  Constant1/1 -> MATLAB Function2/1(T)
  Constant4/1 -> MATLAB Function2/6(r)
  MATLAB Function2/1(u1) -> Delay1/1
  MATLAB Function2/2(u2) -> Memory/1

== system NavV1_0421_2017a/Sensor_Data_Process/baro_Data_Process/reinit_baro0 ==
  QGC_sensor_reinit : Inport
  Data : Inport  Port=2
  Detect Increase : simulink/Logic and Bit Operations/Detect Increase  vinit=0.0  OutDataTypeStr=boolean
  Switch : Switch  Criteria=u2 > Threshold
  Unit Delay : UnitDelay  SampleTime=-1  HasFrameUpgradeWarning=on
  dataout : Outport
  wires:
  Unit Delay/1 -> Switch/3
  Data/1 -> Switch/1
  Switch/1 -> dataout/1, Unit Delay/1
  Detect Increase/1 -> Switch/2
  QGC_sensor_reinit/1 -> Detect Increase/1

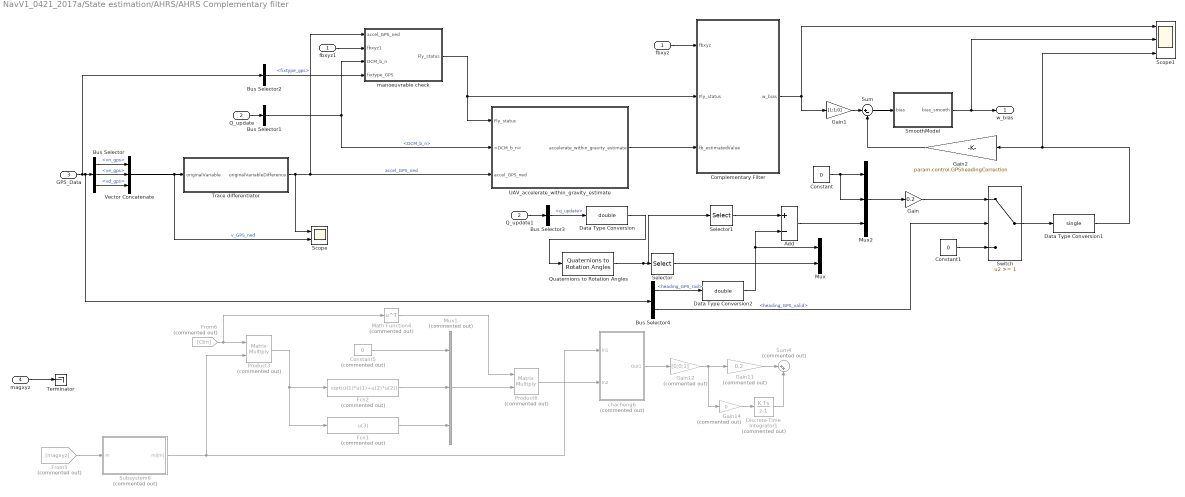
== system NavV1_0421_2017a/State estimation/AHRS/AHRS Complementary filter ==
  fbxyz : Inport
  Q_update : Inport  Port=2
  GPS_Data : Inport  Port=3
  magxyz : Inport  Port=4
  Add : Sum  Inputs=+-
  Bus Selector : BusSelector  OutputSignals=vn_gps,ve_gps,vd_gps
  Bus Selector1 : BusSelector  OutputSignals=DCM_b_n
  Bus Selector2 : BusSelector  OutputSignals=fixtype_gps
  Bus Selector3 : BusSelector  OutputSignals=q_update
  Bus Selector4 : BusSelector  OutputSignals=heading_GPS_rad,heading_GPS_valid
  Complementary Filter : Subsystem
  Constant : Constant  Value=0
  Constant1 : Constant  Value=0
  Constant5 : Constant  Commented=on  Value=0
  Data Type Conversion : DataTypeConversion  OutDataTypeStr=double
  Data Type Conversion1 : DataTypeConversion  OutDataTypeStr=single
  Data Type Conversion2 : DataTypeConversion  OutDataTypeStr=double
  Discrete-Time Integrator1 : DiscreteIntegrator  Commented=on  gainval=1  InitialConditionSetting=State (most efficient)  SampleTime=-1  ICPrevOutput=DiscIntNeverNeededParam  ICPrevScaledInput=DiscIntNeverNeededParam
  Fcn1 : Fcn  Commented=on  Expr=u(3)
  Fcn2 : Fcn  Commented=on  Expr=sqrt(u(1)*u(1)+u(2)*u(2))
  From5 : From  Commented=on  GotoTag=magxyz
  From6 : From  Commented=on  GotoTag=Cbn
  Gain : Gain  Gain=0.2
  Gain1 : Gain  Gain=[1;1;0]
  Gain11 : Gain  Commented=on  Gain=0.2
  Gain12 : Gain  Commented=on  Gain=[0;0;1]
  Gain14 : Gain  Commented=on  Gain=0
  Gain2 : Gain  Gain=param.control.GPSheadingCorrection
  Math Function4 : Math  Commented=on  Operator=transpose  SaturateOnIntegerOverflow=on
  Mux : Mux  Inputs=2
  Mux1 : Mux  Commented=on  Inputs=3
  Mux2 : Mux  Inputs=3
  Product3 : Product  Commented=on  Multiplication=Matrix(*)  SaturateOnIntegerOverflow=on  OutDataTypeStr=Inherit: Same as first input
  Product6 : Product  Commented=on  Multiplication=Matrix(*)  SaturateOnIntegerOverflow=on  OutDataTypeStr=Inherit: Same as first input
  Q_update1 : InportShadow  Port=2
  Quaternions to Rotation Angles : sharedtransform/Quaternions to Rotation Angles  rotationOrder=ZYX
      settings: SourceProductBaseCode=AE,PW,DR,MT,UV,VE
  Scope : Scope  NumInputPorts=2
  Scope1 : Scope  NumInputPorts=3
  Selector : Selector  InputPortWidth=3  IndexOptions=Index vector (dialog)  Indices=[2 3]  OutputSizes=1
  Selector1 : Selector  InputPortWidth=3  IndexOptions=Index vector (dialog)  Indices=[1]  OutputSizes=1
  SmoothModel : Subsystem
  Subsystem6 : Subsystem  Commented=on
  Sum : Sum  Inputs=|+-
  Sum4 : Sum  Commented=on  Inputs=|++
  Switch : Switch  Threshold=1
  Terminator : Terminator
  Trace differentiator : Subsystem
  UAV_accelerate_within_gravity_estimate : Subsystem
  Vector Concatenate : Concatenate  NumInputs=3
  chacheng6 : Subsystem  Commented=on
  fbxyz1 : InportShadow
  manoeuvrable check : Subsystem
  w_bias : Outport
  wires:
  Gain14/1 -> Discrete-Time Integrator1/1
  From6/1 -> Product3/1, Math Function4/1
  Subsystem6/1(m/|m|) -> Product3/2, chacheng6/1(In1)
  Discrete-Time Integrator1/1 -> Sum4/2
  Gain11/1 -> Sum4/1
  Gain12/1 -> Gain11/1, Gain14/1
  Product6/1 -> chacheng6/2(In2)
  Fcn1/1 -> Mux1/3
  From5/1 -> Subsystem6/1(m)
  Math Function4/1 -> Product6/1
  Fcn2/1 -> Mux1/2
  Mux1/1 -> Product6/2
  Constant5/1 -> Mux1/1
  Product3/1 -> Fcn1/1, Fcn2/1
  chacheng6/1(Out1) -> Gain12/1
  GPS_Data/1 -> Bus Selector2/1, Bus Selector4/1, Bus Selector/1
  Bus Selector/1 -> Vector Concatenate/1  "<vn_gps>"
  Bus Selector/2 -> Vector Concatenate/2  "<ve_gps>"
  Bus Selector/3 -> Vector Concatenate/3  "<vd_gps>"
  Q_update/1 -> Bus Selector1/1
  Bus Selector1/1 -> UAV_accelerate_within_gravity_estimate/2(<DCM_b_n>), manoeuvrable check/3(DCM_b_n)  "<DCM_b_n>"
  Vector Concatenate/1 -> Scope/2, Trace differentiator/1(originalVariable)  "v_GPS_ned"
  fbxyz/1 -> Complementary Filter/1(fbxyz)
  UAV_accelerate_within_gravity_estimate/1(accelerate_within_gravity_estimate) -> Complementary Filter/3(fb_estimatedValue)
  Trace differentiator/1(originalVariableDifference) -> Scope/1, UAV_accelerate_within_gravity_estimate/3(accel_GPS_ned), manoeuvrable check/1(accel_GPS_ned)  "accel_GPS_ned"
  fbxyz1/1 -> manoeuvrable check/2(fbxyz1)
  Bus Selector2/1 -> manoeuvrable check/4(fixtype_GPS)  "<fixtype_gps>"
  manoeuvrable check/1(Fly_status) -> Complementary Filter/2(Fly_status), UAV_accelerate_within_gravity_estimate/1(Fly_status)
  magxyz/1 -> Terminator/1
  Complementary Filter/1(w_bias) -> Gain1/1, Scope1/1
  Q_update1/1 -> Bus Selector3/1
  Bus Selector3/1 -> Data Type Conversion/1  "<q_update>"
  Data Type Conversion/1 -> Quaternions to Rotation Angles/1
  Bus Selector4/1 -> Data Type Conversion2/1  "<heading_GPS_rad>"
  Quaternions to Rotation Angles/1 -> Selector1/1, Selector/1
  Selector/1 -> Mux/2
  Data Type Conversion2/1 -> Add/2, Mux/1
  Selector1/1 -> Add/1
  Add/1 -> Mux2/3
  Constant/1 -> Mux2/2, Mux2/1
  Mux2/1 -> Gain/1
  Gain/1 -> Switch/1
  Bus Selector4/2 -> Switch/2  "<heading_GPS_valid>"
  Constant1/1 -> Switch/3
  Switch/1 -> Data Type Conversion1/1
  Sum/1 -> SmoothModel/1(bias)
  Data Type Conversion1/1 -> Scope1/3, Gain2/1
  Gain1/1 -> Sum/1
  SmoothModel/1(bias_smooth) -> Scope1/2, w_bias/1
  Gain2/1 -> Sum/2

== system NavV1_0421_2017a/State estimation/AHRS/Init_Q0 ==
  U : Inport
  accl_B_m/s_LPF : Inport  Port=2
  Magn_B_guess_LPF : Inport  Port=3
  Constant : Constant  Value=[1 0 0 0]  OutDataTypeStr=single
  Constant1 : Constant
  Detect Increase : simulink/Logic and Bit Operations/Detect Increase  vinit=0.0  OutDataTypeStr=boolean
  Horizontal_attitude : Subsystem  TreatAsAtomicUnit=on
  Scope : Scope
  Scope1 : Scope
  Switch : Switch  Criteria=u2 > Threshold
  Switch1 : Switch  Criteria=u2 > Threshold
  quat_0 : Outport
  wires:
  Detect Increase/1 -> Scope/1, Switch1/2, Horizontal_attitude/Enable
  Magn_B_guess_LPF/1 -> Horizontal_attitude/2(Magn_B_guess_LPF)
  U/1 -> Detect Increase/1
  accl_B_m/s_LPF/1 -> Horizontal_attitude/1(accl_B_m/s_LPF)
  Switch1/1 -> Scope1/1, Switch/2, Switch1/3
  Constant1/1 -> Switch1/1
  Switch/1 -> quat_0/1
  Constant/1 -> Switch/3
  Horizontal_attitude/1(quat_0) -> Switch/1

== system NavV1_0421_2017a/State estimation/AHRS/att_update ==
  Sensor_data : Inport
  quat_0 : Inport  Port=2  PortDimensions=4
  init_flag : Inport  Port=3
  wbias : Inport  Port=4  PortDimensions=3
  Add : Sum
  Bus Creator : BusCreator  Inputs=2
  Bus Selector1 : BusSelector  OutputSignals=IMU_Data.gyro_B_rad/s_LPF
  Bus Selector2 : BusSelector  OutputSignals=GPS_Data.heading_GPS_rad,GPS_Data.heading_GPS_valid
  Delay : Delay  DelayLength=1  InitialConditionSource=Input port  ExternalReset=Level hold
      settings: InputPortMap=u0,r5,p4
  Detect Increase : simulink/Logic and Bit Operations/Detect Increase  vinit=0.0  OutDataTypeStr=boolean
  Gain : Gain  Gain=dt
  Memory : Memory  X0=zeros(3,1)
  QuatMult : MATLAB Function  TreatAsAtomicUnit=on
  Quaternions to Direction Cosine Matrix : sharedtransform/Quaternions to  Direction Cosine Matrix
      settings: SourceProductBaseCode=AE,PW,DR,MT,UV,VE
  Sensor_data1 : InportShadow
  Transpose : Math  Operator=transpose  SaturateOnIntegerOverflow=on
  rv2q : MATLAB Function  TreatAsAtomicUnit=on
  uniformization : Subsystem
  att_update : Outport
  wires:
  rv2q/1(quaternion) -> QuatMult/2(quatB)
  Add/1 -> Gain/1
  uniformization/1(Q o) -> Delay/1, Bus Creator/1, Quaternions to Direction Cosine Matrix/1  "q_update"
  Bus Selector1/1 -> Add/1  "<gyro_B_rad/s_LPF>"
  Gain/1 -> rv2q/1(rotVec)  "correctedDelAng"
  Sensor_data/1 -> Bus Selector1/1
  QuatMult/1(quatOut) -> uniformization/1(Q i)
  Delay/1 -> QuatMult/1(quatA)
  quat_0/1 -> Delay/3
  Quaternions to Direction Cosine Matrix/1 -> Transpose/1
  Transpose/1 -> Bus Creator/2  "DCM_b_n"
  Bus Creator/1 -> att_update/1
  init_flag/1 -> Detect Increase/1
  Detect Increase/1 -> Delay/2
  wbias/1 -> Memory/1
  Sensor_data1/1 -> Bus Selector2/1
  Bus Selector2/1 -> ?  "<heading_GPS_rad>"
  Memory/1 -> Add/2

== system NavV1_0421_2017a/State estimation/Translation_estimate/High data source selection ==
  note: 气压计、激光雷达、GPS三种测量高度模式
      | 选择依据：
      | 激光雷达>GPS>气压计
      | 当相对高度在20m内且TOFIns > H0，优先使用TOF
  Sensor_data : Inport
  Bus Selector1 : BusSelector  OutputSignals=GPS_Data.fixtype_gps,TOF_Data.TOF_sts,TOF_Data.TOF_Inten,TOF_Data.H_TOF_TD
  Compare To Constant : simulink/Logic and Bit Operations/Compare To Constant  relop=>=  const=1  OutDataTypeStr=boolean
  Compare To Constant1 : simulink/Logic and Bit Operations/Compare To Constant  relop=>=  const=1  OutDataTypeStr=boolean
  Compare To Constant2 : simulink/Logic and Bit Operations/Compare To Constant  relop=>=  const=100  OutDataTypeStr=boolean
  Compare To Constant3 : simulink/Logic and Bit Operations/Compare To Constant  relop=<=  const=20  OutDataTypeStr=boolean
  Compare To Constant4 : simulink/Logic and Bit Operations/Compare To Constant  relop=>=  const=0.5  OutDataTypeStr=boolean
  Logical Operator : Logic  Inputs=4  AllPortsSameDT=off  OutDataTypeStr=boolean
  Logical Operator1 : Logic  Operator=NOT  Inputs=3  AllPortsSameDT=off  OutDataTypeStr=boolean
  Logical Operator2 : Logic  AllPortsSameDT=off  OutDataTypeStr=boolean
  HTOF_vaild_flag : Outport
  HGPS_vaild_flag : Outport  Port=2
  wires:
  Logical Operator/1 -> HTOF_vaild_flag/1, Logical Operator1/1
  Bus Selector1/3 -> Compare To Constant2/1  "<TOF_Inten>"
  Compare To Constant3/1 -> Logical Operator/3
  Logical Operator1/1 -> Logical Operator2/2
  Logical Operator2/1 -> HGPS_vaild_flag/1
  Compare To Constant/1 -> Logical Operator2/1
  Bus Selector1/2 -> Compare To Constant1/1  "<TOF_sts>"
  Bus Selector1/4 -> Compare To Constant4/1, Compare To Constant3/1  "<H_TOF_TD>"
  Compare To Constant2/1 -> Logical Operator/2
  Compare To Constant1/1 -> Logical Operator/1
  Bus Selector1/1 -> Compare To Constant/1  "<fixtype_gps>"
  Sensor_data/1 -> Bus Selector1/1
  Compare To Constant4/1 -> Logical Operator/4

== system NavV1_0421_2017a/State estimation/Translation_estimate/Rxy_Horizontal_estimation ==
  Vn : Inport
  Enable : Inport  Port=2
  Sensor_data2 : Inport  Port=3
  Add1 : Sum  Inputs=+-
  Bus Selector1 : BusSelector  OutputSignals=GPS_Data.pos_N_gps,GPS_Data.pos_E_gps
  Delay1 : Delay  DelayLength=1
  Integrator_R_Horizontal : Subsystem
  Mux1 : Mux  Inputs=2
  Rxy_kalman filter2 : Subsystem  mask{F=diag([-0.1,-0.1,-0.01,-0.01]), H=[1,0,-1,0;0,1,0,-1], Q=diag([1,1,0.1,0.1]), R=diag([0.1,0.1]), P0=diag([0.8,0.8,0.5,0.5])}
      mask prompts: F "状态转移矩阵：F"; H "观测转移矩阵：H"; Q "预测噪声协方差矩阵：Q"; R "量测噪声协方差矩阵：R"; P0 "初始协方差矩阵：P0"
      mask DialogControl DescTextVar Prompt: Kalman Filter
  Scope1 : Scope  NumInputPorts=2
  Selector1 : Selector  InputPortWidth=4  IndexOptions=Index vector (dialog)  Indices=[1 2]  OutputSizes=1
  R_n&e : Outport
  wires:
  Selector1/1 -> Integrator_R_Horizontal/2(dR)
  Mux1/1 -> Add1/2, Scope1/2
  Delay1/1 -> Selector1/1, Rxy_kalman filter2/1(X)
  Sensor_data2/1 -> Integrator_R_Horizontal/3(Sensor_data2), Bus Selector1/1
  Bus Selector1/2 -> Mux1/2  "<pos_E_gps>"
  Integrator_R_Horizontal/1(R_n&e) -> R_n&e/1, Scope1/1, Add1/1
  Bus Selector1/1 -> Mux1/1  "<pos_N_gps>"
  Enable/1 -> Rxy_kalman filter2/3(Enable)
  Rxy_kalman filter2/1(XOut) -> Delay1/1
  Add1/1 -> Rxy_kalman filter2/2(Z)
  Vn/1 -> Integrator_R_Horizontal/1(Vn)

== system NavV1_0421_2017a/State estimation/Translation_estimate/Subsystem ==
  note: Hd to H
  Vh_vertical_eastimate : Inport
  sensor_data : Inport  Port=2
  Vertical_vaild_flag : Inport  Port=3
  Add : Sum  Inputs=++--
  Bus Selector : BusSelector  OutputSignals=QGC_sensor_reinit,TOF_Data.H_TOF_TD,GPS_Data.pos_D_gps
  Bus Selector1 : BusSelector  OutputSignals=HTOF_vaild,HGPS_vaild
  Delay : Delay  DelayLength=1  InitialConditionSource=Input port  ExternalReset=Level hold
      settings: InputPortMap=u0,r5,p4
  Gain : Gain  Gain=-1
  Gain1 : Gain  Gain=dt  SaturateOnIntegerOverflow=on  OutDataTypeStr=Inherit: Same as input  ParamDataTypeStr=Inherit: Same as input
  Scope : Scope  NumInputPorts=3
  VH_correctionbyTOF : Subsystem
  VH_correctionbyTOF1 : Subsystem
  H_estimation : Outport
  wires:
  sensor_data/1 -> Bus Selector/1
  Bus Selector1/1 -> VH_correctionbyTOF/Enable  "<HTOF_vaild>"
  Vh_vertical_eastimate/1 -> Gain1/1
  Bus Selector/3 -> Gain/1  "<pos_D_gps>"
  Bus Selector1/2 -> VH_correctionbyTOF1/Enable  "<HGPS_vaild>"
  Bus Selector/1 -> Delay/2  "<QGC_sensor_reinit>"
  Vertical_vaild_flag/1 -> Bus Selector1/1
  VH_correctionbyTOF1/1(H_correctionbyGPS) -> Add/4
  Bus Selector/2 -> Scope/1, VH_correctionbyTOF/2(<H_TOF_m/s_TD>)  "<H_TOF_TD>"
  Gain1/1 -> Add/1
  Delay/1 -> Add/2
  VH_correctionbyTOF/1(H_correctionbyTOF) -> Add/3
  Gain/1 -> VH_correctionbyTOF1/2(H_gps), Scope/2, Delay/3
  Add/1 -> Scope/3, H_estimation/1, VH_correctionbyTOF/1(H_k_1), VH_correctionbyTOF1/1(H_k_1), Delay/1

== system NavV1_0421_2017a/State estimation/Translation_estimate/V_Horizontal_estimation ==
  An : Inport
  Sensor_data2 : Inport  Port=2
  Add : Sum  Inputs=+-
  Bus Selector2 : BusSelector  OutputSignals=GPS_Data.vn_gps,GPS_Data.ve_gps
  Delay : Delay  DelayLength=1
  Detect Change : simulink/Logic and Bit Operations/Detect Change  vinit=0  OutDataTypeStr=boolean
  Integrator_V_Horizontal : Subsystem
  Mux : Mux  Inputs=2
  Rxy_kalman filter1 : Subsystem  mask{F=diag([-0.1,-0.1,-0.01,-0.01]), H=[1,0,-1,0;0,1,0,-1], Q=diag([1,1,0.1,0.1]), R=diag([0.1,0.1]), P0=diag([0.8,0.8,0.5,0.5])}
      mask prompts: F "状态转移矩阵：F"; H "观测转移矩阵：H"; Q "预测噪声协方差矩阵：Q"; R "量测噪声协方差矩阵：R"; P0 "初始协方差矩阵：P0"
      mask DialogControl DescTextVar Prompt: Kalman Filter
  Scope : Scope  NumInputPorts=2
  Selector : Selector  InputPortWidth=4  IndexOptions=Index vector (dialog)  Indices=[1 2]  OutputSizes=1
  vxy_estimout : Outport
  V_n&e : Outport  Port=2
  GPS_v_enable : Outport  Port=3
  wires:
  Delay/1 -> Selector/1, Rxy_kalman filter1/1(X)
  Selector/1 -> Integrator_V_Horizontal/2(dv)
  Bus Selector2/1 -> Detect Change/1, Mux/1  "<vn_gps>"
  Mux/1 -> Scope/2, Add/2
  Bus Selector2/2 -> Mux/2  "<ve_gps>"
  Rxy_kalman filter1/1(XOut) -> Delay/1
  Integrator_V_Horizontal/1(V_n&e) -> V_n&e/1, vxy_estimout/1, Scope/1, Add/1
  Detect Change/1 -> GPS_v_enable/1, Rxy_kalman filter1/3(Enable)
  Add/1 -> Rxy_kalman filter1/2(Z)
  An/1 -> Integrator_V_Horizontal/1(An)
  Sensor_data2/1 -> Bus Selector2/1, Integrator_V_Horizontal/3(Sensor_data2)
